simulink model "pospolix_rigido"  (R2020b)
settings: Solver=VariableStepAuto  StartTime=0.0  StopTime=3  RelTol=1e-3
values from neighbouring files (symbols this model uses):
  m = config_dc(parx)    [main.m]
  parx = parametri()    [main.m]
  pp_c = pos_poli_cc_x(m, ac,2)    [main.m]
  pp_m = pos_poli_cc_x(m, ac,1)    [main.m]
undefined symbols (not defined in the file or in its folder): Evaluate_Trajectory
settings Model: Creator=stefa  LastModifiedBy=user
settings DebuggingCC: AlgebraicLoopMsg=none  SFMachineParentedDataDiag=error

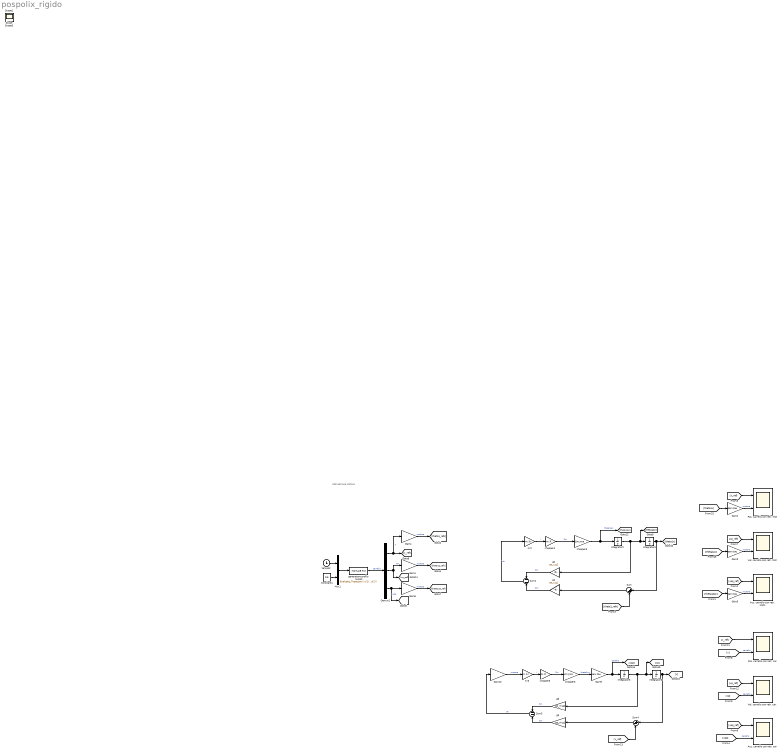
== system pospolix_rigido ==
  note: Retroazione Motore
  Acc. carrello con retr. Mot1 : Scope  NumInputPorts=2
  Acc. carrello con retr. car : Scope  NumInputPorts=2
  Constant1 : Constant  Value=0.6
  Demux2 : Demux  Outputs=3
  Gain{1,4,6,10} (4 alike) : Gain  Gain=1/parx.tau
  Gain{2..3,5,9} (4 alike) : Gain  Gain=parx.tau
  Integrator{2..3,5..6} (4 alike) : Integrator
  Kr2 : Gain  Gain=m.kr
  Kr3 : Gain  Gain=m.kr
  Mux1 : Mux  Inputs=2
  Pos. carrello con retr. Mot : Scope  NumInputPorts=2
  Pos. carrello con retr. car : Scope  NumInputPorts=2
  Sum : Sum  Inputs=|+-
  Sum2 : Sum  Inputs=--
  Sum4 : Sum  Inputs=|+-
  Sum5 : Sum  Inputs=--
  Vel. carrello con retr. Mot : Scope  NumInputPorts=2
  Vel. carrello con retr. car. : Scope  NumInputPorts=2
  chopper3 : Gain  Gain=1/m.Jma
  chopper4 : Gain  Gain=m.K
  chopper5 : Gain  Gain=1/m.Jma
  chopper6 : Gain  Gain=m.K
  g1 : Gain  Gain=pp_c.g1
  g2 : Gain  Gain=pp_c.g2
  g5 : Gain  Gain=pp_m.g1
  g6 : Gain  Gain=pp_m.g2
  generatore profilo moto2 : MATLABFcn  MATLABFcn=Evaluate_Trajectory( u(1) , u(2))  OutputDimensions=3
  tempo2 : Clock
  Scope : Scope
  Scope1 : Scope
  Scope3 : Scope
  wires:
  Mux1/1 -> generatore profilo moto2/1
  generatore profilo moto2/1 -> Demux2/1  "carrello"
  Constant1/1 -> Mux1/2
  tempo2/1 -> Mux1/1
  Demux2/1 -> [x_ref], Gain4/1  "X"
  Demux2/2 -> Gain1/1, [xp_ref]  "XP"
  [xp_ref] -> Vel. carrello con retr. Mot/1
  [x_ref] -> Pos. carrello con retr. Mot/1
  Gain1/1 -> [theta1p_refx]  "motore"
  Gain4/1 -> [theta1_refx]  "motore"
  [theta1x] -> Gain2/1
  [theta1px] -> Gain3/1
  Gain3/1 -> Vel. carrello con retr. Mot/2  "motore"
  Gain2/1 -> Pos. carrello con retr. Mot/2  "motore"
  [theta1ppx] -> Gain5/1
  Gain5/1 -> Acc. carrello con retr. Mot1/2  "motore"
  [xpp_ref] -> Acc. carrello con retr. Mot1/1
  Demux2/3 -> Gain6/1, [xpp_ref]  "XPP"
  Gain6/1 -> [theta1pp_refx]  "motore"
  Kr2/1 -> chopper4/1  "I"
  Integrator3/1 -> Sum/1, [theta1x]
  chopper3/1 -> [theta1ppx], Integrator2/1  "theta1px"
  chopper4/1 -> chopper3/1  "Cm"
  Sum2/1 -> Kr2/1  "Va"
  Integrator2/1 -> g2/1, [theta1px], Integrator3/1
  Sum/1 -> g1/1
  [theta1_refx] -> Sum/2
  g2/1 -> Sum2/1  "Cm"
  g1/1 -> Sum2/2  "Cm"
  [x] -> Pos. carrello con retr. car/2  "carrello"
  [xpp] -> Acc. carrello con retr. car/2  "carrello"
  [xpp_ref] -> Acc. carrello con retr. car/1
  [xp] -> Vel. carrello con retr. car./2  "carrello"
  [xp_ref] -> Vel. carrello con retr. car./1
  [x_ref] -> Pos. carrello con retr. car/1
  Gain9/1 -> Integrator5/1, [xpp]  "carrello"
  Gain10/1 -> Kr3/1  "motore"
  Integrator6/1 -> Sum4/1, [x]
  g5/1 -> Sum5/2  "Cm"
  Kr3/1 -> chopper6/1  "I"
  Integrator5/1 -> g6/1, [xp], Integrator6/1
  chopper6/1 -> chopper5/1  "Cm"
  g6/1 -> Sum5/1  "Cm"
  Sum4/1 -> g5/1
  Sum5/1 -> Gain10/1  "Va"
  [x_ref] -> Sum4/2
  chopper5/1 -> Gain9/1  "theta1px"
